simulink library "m3_common_lib"  (R2021b)
settings: Solver=ode45  StartTime=0.0  StopTime=10.0  RelTol=1e-3
undefined symbols (not defined in the file or in its folder): ACCEL_PRE_MULT, APDT_SrvcMgr_IRVHVDCSubFcnReq, C_C1GearNumbers, C_C1GearRatios, C_Calibration, C_DitherWaveform, C_GearOffset, C_GearRatioIn, C_GearRatioInverseOut, C_GearRatioOut, CLUTCH_INNER_LOOP_UPDATE_RATE, CONSTANT, DEGRADED_MODE_SIZE, Dem_EventStatusType, DiscIntNeverNeededParam, F_FAULT_ENUM, F_NOFAULT, F_OUTOFRANGE, F_RATELIMIT, FALSE, FMI14_SPECIAL_INSTRUCTIONS, FMI20_DATA_DRIFTED_HIGH, FMI21_DATA_DRIFTED_LOW, FMI29_RESERVED_FOR_SAE_ASSIGNMENT, FMI30_RESERVED_FOR_SAE_ASSIGNMENT, FMI31_CONDITION_EXISTS, FMI32_NO_FAULT, IC, k_accel, k_mean, MAX_UINT32, MEAN_PRE_MULT, NTriggers, QLTY_SIGNAL_FAILED, QLTY_SIGNAL_FULLY_FUNCTION, QLTY_SIGNAL_SUBSTITUTED_BY_1ST_CHOICE, QLTY_SIGNAL_SUBSTITUTED_BY_2ND_CHOICE, QLTY_SIGNAL_SUBSTITUTED_BY_3RD_CHOICE, QLTY_SIGNAL_SUBSTITUTED_BY_4TH_CHOICE, SAMPLE_TIME_100us, simin, T_TestPoint, TF_FALSE, TF_TRUE, TimeStep, TRUE, WORKSPACE_UPDATE_RATE, Zero, ZERO
libraries: $bdroot x121, simulink x23, simulink_extras x4, MBD_EPS_Local_Blockset x4
(part 1 of 10)
Description:
  | Common library
  | 
  | 
  | 
  | 
  | 
  | 
  | 
  | 
  | 
  | 
  | 
  | 
  | 
  | 
  | 
  | 
  | 
  | 
  | 
  | 
  | 
  | 
  | 
  | 
  | 
  | 
  | 
  | 
  | 
  | 
  | 
  | 
  | 
  | 
  | 
  | 
  | 
  | 
  | 
  | 
  | 
  | 
  | Utility functions useful for embedded control applications.
settings Model: Creator=George Brunemann  LastModifiedBy=E0644758
settings Model: ModifiedComment=|
  | E0072681 -- Fri Jan 08 10:38:41 2010 -- Version 2.15
  | Merged change to cmd-fbk block
settings Model: ModifiedHistory=|
  | E0072681 -- Fri Jan 08 10:38:41 2010 -- Version 2.15
  | Merged change to cmd-fbk block
  | 
  | E0072681 -- Fri Jan 08 10:38:41 2010 -- Version 2.15
  | Merged change to cmd-fbk block
  | 
  | E0072681 -- Fri Jan 08 10:38:27 2010 -- Version 2.14
  | 
  | 
  | E0072118 -- Tue Jan 05 16:47:56 2010 -- Version 2.13
  | 
  | 
  | E0072118 -- Tue Jan 05 16:43:14 2010 -- Version 2.12
  | 
  | 
  | E0072118 -- Fri Dec 18 15:21:16 2009 -- Version 2.11
  | 
  | 
  | E0072118 -- Fri Dec 18 11:28:11 2009 -- Version 2.10
  | 
  | 
  | E0072118 -- Fri Dec 18 11:22:41 2009 -- Version 2.9
  | 
  | 
  | E0072118 -- Fri Dec 18 11:10:11 2009 -- Version 2.8
  | 
  | 
  | E0072118 -- Tue Dec 15 11:02:29 2009 -- Version 2.7
  | 
  | 
  | e0072681 -- Fri Nov 20 14:24:13 2009 -- Version 2.6
  | 
  | 
  | e0072681 -- Fri Nov 20 14:05:16 2009 -- Version 2.5
  | 
  | 
  | E0072681 -- Fri Nov 13 14:35:41 2009 -- Version 2.4
  | 
  | 
  | E0072681 -- Fri Nov 13 11:01:17 2009 -- Version 2.3
  | Added new diagnostic blocks
  | 
  | E0072681 -- Tue Oct 27 17:06:03 2009 -- Version 2.2
  | Changed names on ETP and ETPWT
  | 
  | E0072681 -- Tue Oct 27 15:45:40 2009 -- Version 2.1
  | Merged ETP and ETPWT blocks with IC's into Arbiter library
  | 
  | $Author: allison $ -- $Date: 2006/06/13 14:35:43 $ -- Version $Revision: 1.69 $
settings SolverCC: AlgebraicLoopSolver=TrustRegion
settings DataIOCC: LimitDataPoints=on  SaveFormat=Array  SignalLoggingSaveFormat=ModelDataLogs  ReturnWorkspaceOutputs=off
settings OptimizationCC: BlockReduction=off  BooleanDataType=off  ExpressionDepthLimit=2147483647  LifeSpan=inf
settings DebuggingCC: SaveWithParameterizedLinksMsg=none  UnderspecifiedInitializationDetection=Classic  MergeDetectMultiDrivingBlocksExec=none  SignalResolutionControl=TryResolveAllWithWarning  MultiTaskCondExecSysMsg=none  FcnCallInpInsideContextMsg=warning  StateNameClashWarn=warning  SFUnexpectedBacktrackingDiag=warning  SFNoUnconditionalDefaultTransitionDiag=warning  SFExecutionAtInitializationDiag=none  SFMachineParentedDataDiag=warning  ArithmeticOperatorsInVariantConditions=warning
settings HardwareCC: ProdBitPerPointer=32  ProdBitPerSizeT=32  ProdBitPerPtrDiffT=32  ProdLargestAtomicFloat=None  ProdIntDivRoundTo=Undefined  ProdEndianess=Unspecified  ProdWordSize=32  ProdHWDeviceType=32-bit Generic  TargetUnknown=on
settings ModelReferenceCC: PropagateSignalLabelsOutOfModel=off
settings SFSimCC: SimCustomHeaderCode="#include \"DiagDebounce.h\""  SimUserSources=DiagDebounce.c  CustomCodeUndefinedFunction=UseInterfaceOnly
settings RTWCC: RTWUseSimCustomCode=on  CustomHeaderCode="#include \"DiagDebounce.h\""  CustomSource=DiagDebounce.c
settings CodeAppCC: StateflowObjectComments=on
settings GRTTargetCC: TargetLangStandard=C89/C90 (ANSI)  CombineOutputUpdateFcns=off  GRTInterface=on
settings ConfigComp: CovMetricSettings=dw  CovSaveCumulativeToWorkspaceVar=on  CovSaveSingleToWorkspaceVar=on  CovExternalEMLEnable=off

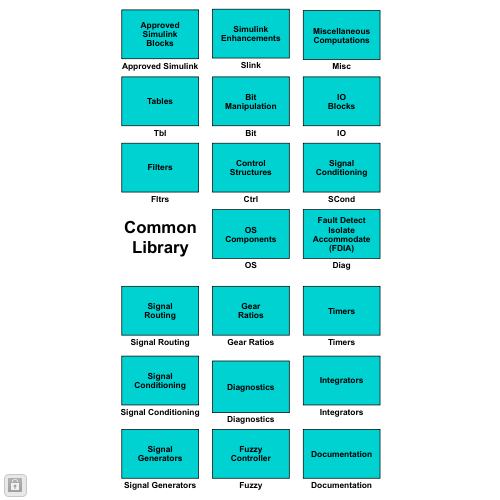
[thumbnail: Simulink's stored preview of the top-level diagram]
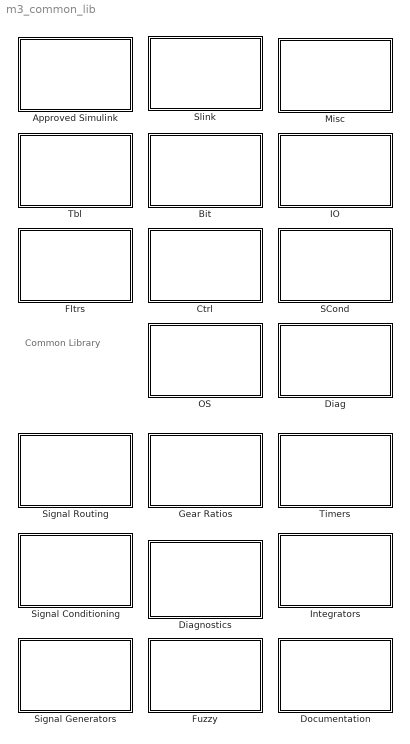
== system m3_common_lib ==
  note: Common
      | Library
  Approved Simulink : Subsystem
      mask Display: disp('Approved\nSimulink\nBlocks')
  Bit : Subsystem
      mask Display: disp('Bit\nManipulation')
  Ctrl : Subsystem
      mask Display: disp('Control\nStructures')
  Diag : Subsystem
      mask Display: disp('Fault Detect\nIsolate\nAccommodate\n(FDIA)')
  Diagnostics : Subsystem
      mask Display: disp('Diagnostics')
  Documentation : Subsystem
      mask Display: disp('Documentation')
  Fltrs : Subsystem
      mask Display: disp('Filters')
  Fuzzy : Subsystem
      mask Display: disp('Fuzzy\nController')
  Gear Ratios : Subsystem
      mask Display: disp('Gear\nRatios')
  IO : Subsystem
      mask Display: disp('IO\nBlocks')
  Integrators : Subsystem
      mask Display: disp('Integrators')
  Misc : Subsystem
      mask Display: disp('Miscellaneous\nComputations')
  OS : Subsystem
      mask Display: disp('OS\nComponents')
  SCond : Subsystem
      mask Display: disp('Signal\nConditioning')
  Signal Conditioning : Subsystem
      mask Display: disp('Signal\nConditioning')
  Signal Generators : Subsystem
      mask Display: disp('Signal\nGenerators')
  Signal Routing : Subsystem
      mask Display: disp('Signal\nRouting')
  Slink : Subsystem
      mask Display: disp('Simulink\nEnhancements')
  Tbl : Subsystem
      mask Display: disp('Tables')
  Timers : Subsystem
      mask Display: disp('Timers')

== system m3_common_lib/Approved Simulink ==
  note: Unit Tested and Approved Simulink Components
  Basic IO : Subsystem
      mask Display: disp('Basic\nInput/Output')
  Discrete And Discontinuities : Subsystem
      mask Display: disp('Discrete')
  Flip Flops : Subsystem
      mask Display: disp('Flip Flops')
  Grouping : Subsystem
      mask Display: disp('Bus and\nMux')
  Math And Logic : Subsystem
      mask Display: disp('Math Operations')
  Signal Attributes : Subsystem
      mask Display: disp('Signal Attributes')
  SubSys Triggers : Subsystem  TreatAsAtomicUnit=on
      mask Display: disp('Subsystem\nEnable and\nTriggers')

== system m3_common_lib/Bit ==
  note: Bit Manipulation
  Bit Operator : Subsystem  mask(CL Bit Operator){Pack=Bit Unpack, DType=UINT8}
      mask prompts: Pack "Binary Operation"; DType "Data Type"
      mask help:
      | Pack or unpack binary data
      |
      | Input and Output vary with mask parameter settings.
      |
      | NgEK, Inc.
      mask init:
      | bit_morph
      mask Help: web(which(['common_lib1.html']))
      mask TypeOptions Pack: Bit Unpack | Bit Pack
      mask TypeOptions DType: UINT8 | UINT16 | UINT32
      mask Display:
      | patch([0.3 0.3 0.7 0.7], [0.35 0.65 0.65 0.35], [255/255 127/255 255/255])
      | disp('Bit\nUnpacker');
      | 
      | port_label('input',1,'Input');
      | port_label('output',1,'Bit 7');
      | port_label('output',2,'Bit 6');
      | port_label('output',3,'Bit 5');
      | port_label('output',4,'Bit 4');
      | port_label('output',5,'Bit 3');
      | port_label('output',6,'Bit 2');
      | port_label('output',7,'Bit 1');
      | port_label('output',8,'Bit 0');
  uint16 Bit Pack : Stateflow chart  TreatAsAtomicUnit=on
  uint16 Bit Unpack : Stateflow chart  TreatAsAtomicUnit=on
  uint8 Bit Pack : Stateflow chart  TreatAsAtomicUnit=on
  uint8 Bit Unpack : Stateflow chart  TreatAsAtomicUnit=on

== system m3_common_lib/Ctrl ==
  note: Control Structures
  Derivative : Subsystem  RTWFcnName=DER  mask(CL Derivative){TimeStep=[]}
      mask prompts: TimeStep "Time Step"
      mask help:
      | Derivative with low pass filtering.  Outputs zero when reset is held, limited to the upper and lower limit inputs.
      |
      | X(1) = input
      | X(2) = low pass cutoff frequency
      | X(3) = upper limit
      | X(4) = lower limit
      | X(5) = reset
      |
      | Y(1) = output
      |
      | Time step is entered via mask parameter.
      | NgEK, Inc.
      mask init:
      | %switch class(TimeStep)
      | % case ('double')
      | %    Zero        = double( 0.0);
      | %    One         = double( 1.0);
      | % case ('single')
      |      Zero        = single( 0.0);
      |      One         = single( 1.0);
      | %end
      | Ts = single(TimeStep);
      settings: RTWFcnNameOpts=User specified  RTWFileNameOpts=Use function name
      mask Help: web(which(['common_lib2.html']))
      mask Display:
      | patch([0.3 0.3 0.7 0.7], [0.35 0.65 0.65 0.35], [255/255 127/255 255/255])
      | disp('Derivative')
      | port_label('input', 1, 'input')
      | port_label('input', 2, 'cutoff')
      | port_label('input', 3, 'ulim')
      | port_label('input', 4, 'llim')
      | port_label('input', 5, 'reset?')
      | port_label('output', 1, 'output')
  Dither : Subsystem  mask(CL Dither){TimeStep=[]}
      mask prompts: TimeStep "Time Step"
      mask help:
      | Output a rectangular dither signal of specified amplitude and frequency.
      | A first order filter of specified time constant is applied to smooth transitions.
      |
      | X(1) = amplitude
      | X(2) = frequency
      | X(3) = filter time constant
      |
      | Y(1) = output
      |
      | Time step is entered via mask parameter.
      | NgEK, Inc.
      mask init:
      | h = [gcb '/Data Type Conversion'];
      | 
      | %switch class(TimeStep)
      | %   case ('double')
      | %      MinusOne    = double(-1.0);
      | %      Zero        = double( 0.0);
      | %      One         = double( 1.0);
      | %      Two         = double( 2.0);
      | %      ZeroFive    = double( 0.5);
      | %      lim         = double(4e-5);
      | %      set_param(h, 'DataType','double');
      | %   case ('single')
      |        MinusOne    = single(-1.0);
      |        Zero        = single( 0.0);
      |        One         = single( 1.0);
      |        Two         = single( 2.0);
      |        ZeroFive    = single( 0.5);
      |        lim         = single(4e-5);
      |        set_param(h, 'DataType','single');
      | %end;
      mask Help: web(which(['common_lib8.html']))
      mask Display:
      | patch([0.375 0.375 0.625 0.625], [0.35 0.65 0.65 0.35], [255/255 127/255 255/255])
      | disp('Dither')
      | port_label('input', 1, 'amplitude')
      | port_label('input', 2, 'frequency')
      | port_label('input', 3, 'tau')
      | port_label('output', 1, 'output')
  Dither w Reset : Subsystem  mask(CL Dither with Reset){TimeStep=[]}
      mask prompts: TimeStep "Time Step"
      mask help:
      | Output a rectangular dither signal of specified amplitude and frequency.
      | A first order filter of specified time constant is applied to smooth transitions.
      |
      | X(1) = amplitude
      | X(2) = frequency
      | X(3) = filter time constant
      |
      | Y(1) = output
      | Y(2) = reset (switched output)
      |
      | Time step is entered via mask parameter.
      | NgEK, Inc.
      mask init: same as m3_common_lib/Ctrl/Dither
      mask Help: web(which(['common_lib9.html']))
      mask Display:
      | patch([0.375 0.375 0.625 0.625], [0.35 0.65 0.65 0.35], [255/255 127/255 255/255])
      | disp('Dither')
      | port_label('input', 1, 'amplitude')
      | port_label('input', 2, 'frequency')
      | port_label('input', 3, 'tau')
      | port_label('output', 1, 'output')
      | port_label('output', 2, 'reset')
  Integrator : Subsystem  TreatAsAtomicUnit=on  RTWFcnName=INTEGRATOR  mask(CL Integrator){TimeStep=SAMPLE_TIME_100us, IC=single(0)}
      mask prompts: TimeStep "Time Step"; IC "Initial Condition"
      mask help:
      | Determine the integral of the input.
      | If reset is true (1), the integrator is set to the reset condition input.
      |
      | X(1) = input
      | X(2) = upper limit
      | X(3) = lower limit
      | X(4) = reset condition
      | X(5) = reset
      |
      | Y(1) = output
      |
      | Time step is entered via mask parameter.
      | Initial condition is entered via mask parameter.
      |
      | NgEK, Inc.
      settings: RTWFcnNameOpts=User specified  RTWFileNameOpts=Use function name
      mask Help: web(which(['common_lib3.html']))
      mask Display:
      | patch([0.3 0.3 0.7 0.7], [0.35 0.65 0.65 0.35], [255/255 127/255 255/255])
      | disp('Integrator')
      | port_label('input', 1, 'input')
      | port_label('input', 2, 'ulim')
      | port_label('input', 3, 'llim')
      | port_label('input', 4, 'reset_cond')
      | port_label('input', 5, 'reset?')
      | port_label('output', 1, 'output')
  PIDgov : Subsystem  mask(CL PID Governor){TimeStep=, MaxInt=, MinInt=, MaxDrv=, MinDrv=, Tol=, IC=}
      mask prompts: TimeStep "Time Step"; MaxInt "Maximum Integrator Value"; MinInt "Minimum Integrator Value"; MaxDrv "Maximum Derivative Value"; MinDrv "Minimum Derivative Value"; Tol "Tolerance"; IC "Initial Condition"
      mask help:
      | Proportional, integral, and derivative governor with anti-windup.
      | Reset sets integral to zero.
      |
      | X(1) = input
      | X(2) = proportional gain
      | X(3) = integral gain
      | X(4) = derivative gain
      | X(5) = low pass cutoff frequency
      | X(6) = controller output upper limit
      | X(7) = controller output lower limit
      | X(8) = reset
      |
      | Y(1) = output
      |
      | Min and max integrator and derivative limits are entered via mask.
      | Time step is entered via mask parameter.
      | Tolerance for detecting saturation is entered via mask.
      | Initial condition is entered via mask.
      |
      | NgEK, Inc.
      mask init:
      | %switch class(TimeStep)
      | %   case ('double')
      | %      Zero        = double( 0.0);
      | %   case ('single')
      |        Zero        = single( 0.0);
      | %end;
      mask Help: web(which(['common_lib6.html']))
      mask Display:
      | patch([0.35 0.35 0.65 0.65], [0.4 0.6 0.6 0.4], [255/255 127/255 255/255])
      | disp('PID gov')
      | port_label('input', 1, 'error')
      | port_label('input', 2, 'p_gain')
      | port_label('input', 3, 'i_gain')
      | port_label('input', 4, 'd_gain')
      | port_label('input', 5, 'cutoff')
      | port_label('input', 6, 'ulim')
      | port_label('input', 7, 'llim')
      | port_label('input', 8, 'reset?')
      | port_label('output', 1, 'output')
  PIDgov w Preset : Subsystem  mask(CL PID Governor with Preset){TimeStep=0.010, MaxInt=1000, MinInt=-1000, MaxDrv=1000, MinDrv=-1000, Tol=1e-6, IC=0.0}
      mask prompts: TimeStep "Time Step"; MaxInt "Maximum Integrator Value"; MinInt "Minimum Integrator Value"; MaxDrv "Maximum Derivative Value"; MinDrv "Minimum Derivative Value"; Tol "Tolerance"; IC "Initial Condition"
      mask help:
      | Proportional plus Integral Governor with anti-windup and integrator preset.
      |
      | Preset sets output to "preset" and resets integrator to achieve that output.
      | Reset sets integral and output to zero.
      |
      | X(1) = input
      | X(2) = proportional gain
      | X(3) = integral gain
      | X(4) = derivative gain
      | X(5) = low pass cutoff frequency
      | X(6) = controller output upper limit
      | X(7) = controller output lower limit
      | X(8) = preset value
      | X(9) = preset
      | X(10) = reset
      |
      | Y(1) = output
      |
      | Min and max integrator and derivative limits are entered via mask.
      | Time step is entered via mask parameter.
      | Tolerance for detecting saturation is entered via mask.
      | Initial condition is entered via mask.
      |
      | NgEK, Inc.
      mask init:
      | %switch class(TimeStep)
      | %   case ('double')
      | %      Zero        = double( 0.0);
      | %   case ('single')
      |        Zero        = single( 0.0);
      | %end;
      mask Help: web(which(['common_lib7.html']))
      mask Display:
      | patch([0.35 0.35 0.65 0.65], [0.4 0.6 0.6 0.4], [255/255 127/255 255/255])
      | disp('PID gov')
      | port_label('input', 1, 'error')
      | port_label('input', 2, 'p_gain')
      | port_label('input', 3, 'i_gain')
      | port_label('input', 4, 'd_gain')
      | port_label('input', 5, 'cutoff')
      | port_label('input', 6, 'ulim')
      | port_label('input', 7, 'llim')
      | port_label('input', 8, 'preset')
      | port_label('input', 9, 'preset?')
      | port_label('input', 10, 'reset?')
      | port_label('output', 1, 'output')
  PIgov : Subsystem  mask(CL PI Governor){TimeStep=, MaxInt=, MinInt=, Tol=, IC=}
      mask prompts: TimeStep "Time Step"; MaxInt "Maximum Integrator Value"; MinInt "Minimum Integrator Value"; Tol "Tolerance"; IC "Initial Condition"
      mask help:
      | Proportional plus integral governor with anti-windup.
      | Reset sets integral to zero.
      |
      | X(1) = input
      | X(2) = proportional gain
      | X(3) = integral gain
      | X(4) = controller output upper limit
      | X(5) = controller output lower limit
      | X(6) = reset
      |
      | Y(1) = output
      |
      | Time step for integrator is entered via mask.
      | Min and max integrator limits are entered via mask.
      | Tolerance for detecting saturation is entered via mask.
      | Initial condition is entered via mask.
      |
      | NgEK, Inc.
      mask init:
      | %switch class(TimeStep)
      | %   case ('double')
      | %      Zero        = double( 0.0);
      | %   case ('single')
      |        Zero        = single( 0.0);
      | %end;
      mask Help: web(which(['common_lib4.html']))
      mask Display:
      | patch([0.35 0.35 0.65 0.65], [0.4 0.6 0.6 0.4], [255/255 127/255 255/255])
      | disp('PI gov')
      | port_label('input', 1, 'error')
      | port_label('input', 2, 'p_gain')
      | port_label('input', 3, 'i_gain')
      | port_label('input', 4, 'ulim')
      | port_label('input', 5, 'llim')
      | port_label('input', 6, 'reset?')
      | port_label('output', 1, 'output')
  PIgov w Preset : Subsystem  mask(CL PI Governor with Preset){TimeStep=, MaxInt=, MinInt=, Tol=, IC=}
      mask prompts: TimeStep "Time Step"; MaxInt "Maximum Integrator Value"; MinInt "Minimum Integrator Value"; Tol "Tolerance"; IC "Initial Condition"
      mask help:
      | Proportional plus integral governor with anti-windup and integrator preset.
      |
      | Preset sets output to "preset" and resets integrator to achieve that output.
      | Reset sets integrator and output to zero.
      |
      | X(1) = input
      | X(2) = proportional gain
      | X(3) = integral gain
      | X(4) = controller output upper limit
      | X(5) = controller output lower limit
      | X(6) = output preset
      | X(7) = preset
      | X(8) = reset
      |
      | Y(1) = output
      |
      | Time step for integrator is entered via mask.
      | Min and max integrator limits are entered via mask.
      | Tolerance for detecting saturation is entered via mask.
      | Initial condition is entered via mask.
      |
      | NgEK, Inc.
      mask init:
      | %switch class(TimeStep)
      | %   case ('double')
      | %      Zero        = double( 0.0);
      | %   case ('single')
      |        Zero        = single( 0.0);
      | %end;
      mask Help: web(which(['common_lib5.html']))
      mask Display:
      | patch([0.35 0.35 0.65 0.65], [0.4 0.6 0.6 0.4], [255/255 127/255 255/255])
      | disp('PI gov')
      | port_label('input', 1, 'error')
      | port_label('input', 2, 'p_gain')
      | port_label('input', 3, 'i_gain')
      | port_label('input', 4, 'ulim')
      | port_label('input', 5, 'llim')
      | port_label('input', 6, 'preset')
      | port_label('input', 7, 'preset?')
      | port_label('input', 8, 'reset?')
      | port_label('output', 1, 'output')
  Ramp : Subsystem  TreatAsAtomicUnit=on  RTWFcnName=RAMP  mask(CL ramp){TimeStep=[]}
      mask prompts: TimeStep "Time Step"
      mask help:
      | Ramp from A to B over time interval C
      | If reset is true (1), the output is held at the A input.
      |
      | X(1) = starting point for ramp
      | X(2) = ending point for ramp
      | X(3) = time interval for ramp
      | X(4) = reset
      |
      | Y(1) = output
      |
      | Time step is entered via mask parameter.
      |
      | NgEK, Inc.
      mask init:
      | %switch class(TimeStep)
      | %   case ('double')
      | %      Zero        = double( 0.0);
      | %   case ('single')
      |        Zero        = single( 0.0);
      | %end;
      settings: RTWFcnNameOpts=User specified  RTWFileNameOpts=Use function name
      mask Help: web(which(['common_lib50.html']))
      mask Display:
      | patch([0.2 0.2 0.8 0.8], [0.2 0.8 0.8 0.2], [255/255 127/255 255/255])
      | 
      | plot([0.25 0.4 0.6 .75],[.25 .25 .75 .75])
      | 
      | text(.3,.35,'A');text(.65,.65,'B');text(.5,.4,'C')
      | 
      | port_label('input', 1, 'A')
      | port_label('input', 2, 'B')
      | port_label('input', 3, 'C')
      | port_label('input', 4, 'reset?')
      | port_label('output', 1, 'out')
  Subsystem : Subsystem  TreatAsAtomicUnit=on  RTWFcnName=HistogramCntr
      settings: RTWFcnNameOpts=User specified  RTWFileNameOpts=Use function name
  Trajectory : Subsystem  mask(CL Trajectory){TimeStep=, StartRLimIn=, StartRLimOut=, FinalRLimIn=, FinalRLimOut=}
      mask prompts: TimeStep "Time Step"; StartRLimIn "Start Rate Limit Input"; StartRLimOut "Start Rate Limit Output"; FinalRLimIn "Final Rate Limit Input"; FinalRLimOut "Final Rate Limit Output"
      mask help:
      | Control the shape from start_value to final_value using a table of filter tau versus time.
      |
      | The weight stretches the trajectory for values > 1.
      | The weight compresses the trajectory for values <1.
      |
      | X(1)=start_value
      | X(2)=final_value
      | X(3)=weight
      | X(4)=start flag
      |
      | Y(1)=output
      |
      | Update rate, vector of time inputs and tau outputs is entered via mask parameter.
      | NgEK, Inc.
      mask init:
      | %switch class(TimeStep)
      | %   case ('double')
      | %      Zero       = double( 0.0);
      | %      MinusOne   = double(-1.0);
      | %      tol        = double(1e-6);
      | %   case ('single')
      |        Zero       = single( 0.0);
      |        MinusOne   = single(-1.0);
      |        tol       = single(1e-6);
      | %end;
      mask Help: web(which(['common_lib10.html']))
      mask Display:
      | patch([0.4 0.4 0.6 0.6], [0.35 0.65 0.65 0.35], [255/255 127/255 255/255])
      | disp('Traj')
      | port_label('input', 1, 'start_value')
      | port_label('input', 2, 'final_value')
      | port_label('input', 3, 'start_weight')
      | port_label('input', 4, 'final_weight')
      | port_label('input', 5, 'start?')
      | port_label('output', 1, 'output')

== system m3_common_lib/Diag ==
  note: Diagnostics
  CL MinMax Capture : Subsystem  RTWFcnName=MinMaxCap  mask(CL Max Capture){CaptureType=Min, InDataType=single}
      mask prompts: CaptureType "Capture Function"; InDataType "Input DataType"
      mask help:
      | Capture the maximum/minimum value for the input.
      |
      | x(1) = input
      | x(2) = hold?        (hold current max/min value)
      | x(3) = reset?       (reset the output to initial value)
      |
      | y(1) = output
      |
      | The capture function and Input signal datatype are entered via mask parameters.
      |
      | Eaton Controls Engineering COE, 2010.
      mask init:
      | % Change the relational operation and outport label
      | h_input = [gcb '/Relational Operator'];
      | 
      | switch (get_param(gcb,'CaptureType'))
      |     case('Min')
      |        set_param(h_input,'Operator','<');
      |        initvalue = double(999999999999);
      |     case('Max')
      |         set_param(h_input,'Operator','>');
      |         initvalue = double(-999999999999);
      | end;
      | 
      | % Set the Init value to the appropriate value
      | % value for the data type
      | 
      | switch (get_param(gcb,'InDataType'))
      |    case ('double')
      |         InitValue    = double(initvalue);
      |    case ('single')
      |         InitValue    = single(initvalue);
      |    case ('uint32')
      |         InitValue    = uint32(initvalue);
      |    case ('int32')
      |         InitValue    = int32(initvalue);
      |    case ('uint16')
      |         InitValue    = uint16(initvalue);
      |    case ('int16')
      |         InitValue    = int16(initvalue);
      |    case ('uint8')
      |         InitValue    = uint8(initvalue);
      |    case ('int8')
      |         InitValue    = int8(initvalue); 
      | end;
      settings: RTWFcnNameOpts=User specified  RTWFileNameOpts=Use function name
      mask TypeOptions CaptureType: Min | Max
      mask TypeOptions InDataType: double | single | uint32 | int32 | uint16 | int16 | uint8 | int8
      mask Display:
      | patch([0.3 0.3 0.7 0.7],[0.4 0.6 0.6 0.4],[255/255 127/255 255/255])
      | 
      | disp([get_param(gcb,'CaptureType') ' Capture'])
      | 
      | port_label('input', 1, 'input')
      | port_label('input', 2, 'hold?')
      | port_label('input', 3, 'reset?')
      | port_label('output', 1, [get_param(gcb,'CaptureType') ' Value'])
  Command Feedback Test : Subsystem  TreatAsAtomicUnit=on  RTWFcnName=CFT  mask(CL Command Feedback Test){TimeStep=[]}
      mask prompts: TimeStep "Time Step (seconds)"
      mask help:
      | System level check to test if control command is being achieved.
      |
      | During "steady state", check that cmd - fbk  < error_lim
      | Error must occur for error_time seconds before fault is set.
      | Error must not occur for error_time seconds before fault is cleared.
      |
      | "Steady state" is defined as:
      |   command is within tau_lim of filtered command for tau_time
      |
      | NgEK, Inc.
      mask init:
      | %switch class(TimeStep)
      | %   case ('double')
      | %      Zero     = double( 0.0);
      | %      One      = double( 1.0);
      | %      MinusOne = double(-1.0);
      | %   case ('single')
      |        Zero     = single( 0.0);
      |        One      = single( 1.0);
      |        MinusOne = single(-1.0);
      | %end;
      | Ts = single(TimeStep);
      settings: RTWFcnNameOpts=User specified  RTWFileNameOpts=Use function name
      mask Help: web(which(['common_lib11.html']))
      mask Display:
      | patch([0.3 0.3 0.7 0.7], [0.4 0.6 0.6 0.4], [255/255 127/255 255/255]);
      | disp('Cmd-Fbk');
  Fault Counter : Subsystem  RTWFcnName=FLTCNTR  mask(FL Counter){DATATYPE=int16}
      mask prompts: DATATYPE "Counter datatype"
      mask help:
      | Generic fault counter block.
      | Counts up by up_count when fl? is true
      | Counts down by down_count when fl? is false.
      | Sets fc? true if fc_level is reached and clears fc? if zero is reached.
      |
      | X(1) = fault flag
      | X(2) = up count value (positive number)
      | X(3) = down count value (negative number)
      | X(4) = fault code active level
      | X(5) = reset fault code to false and count to zero
      |
      | Y(1) = fault code active flag
      |
      | Initial condition is entered via mask.
      | NgEK, Inc.
      mask init:
      | switch DATATYPE
      |     case (1) %('double')
      |         ZERO     = double(0.0);
      |   case (2) %('single')
      |         ZERO     = single(0.0);
      |   case (3) %('int8')
      |         ZERO     = int8(0.0);
      |     case (4) %('int16')
      |        ZERO     = int16(0.0);
      |    case (5) %('int32')
      |        ZERO     = int32(0.0);
      | end;
      | 
      | strDtype = get_param(gcb,'DATATYPE');
      | %set_param([gcb '/DTC2'],'OutDataTypeStr',strDtype);
      | set_param([gcb '/DTC3'],'OutDataTypeStr',strDtype);
      | %set_param([gcb '/DTC4'],'OutDataTypeStr',strDtype);
      settings: RTWFcnNameOpts=User specified  RTWFileNameOpts=Use function name
      mask Help: web(which(['common_lib49.html']))
      mask TypeOptions DATATYPE: double | single | int8 | int16 | int32
      mask Display:
      | patch([0.35 0.35 0.65 0.65], [0.25 0.75 0.75 0.25], [255/255 127/255 255/255])
      | disp('Fault\nCounter')
      | port_label('input', 1, 'fl?')
      | port_label('input', 2, 'true_count')
      | port_label('input', 3, 'false_count')
      | port_label('input', 4, 'fc_level')
      | port_label('input', 5, 'reset?')
      | port_label('output', 1, 'fc?')
  Fault Counter w Hold : Subsystem  mask(FL Counter){DATATYPE=int16}
      mask prompts: DATATYPE "Counter datatype"
      mask help:
      | Generic fault counter block.
      | Freezes count when hold? is true
      | Counts up by up_count when fl? is true
      | Counts down by down_count when fl? is false.
      | Sets fc? true if fc_level is reached and clears fc? if zero is reached.
      |
      | X(1) = fault flag
      | X(2) = hold flag
      | X(3) = up count value (positive number)
      | X(4) = down count value (negative number)
      | X(5) = fault code active level
      | X(6) = reset fault code to false and count to zero
      |
      | Y(1) = fault code active flag
      |
      | Initial condition is entered via mask.
      | NgEK, Inc.
      mask init:
      | switch DATATYPE
      |     case (1) %('double')
      |         ZERO     = double(0.0);
      |   case (2) %('single')
      |         ZERO     = single(0.0);
      |   case (3) %('int8')
      |         ZERO     = int8(0.0);
      |     case (4) %('int16')
      |        ZERO     = int16(0.0);
      |    case (5) %('int32')
      |        ZERO     = int32(0.0);
      | end;
      mask Help: web(which(['common_lib49.html']))
      mask TypeOptions DATATYPE: double | single | int8 | int16 | int32
      mask Display:
      | patch([0.35 0.35 0.65 0.65], [0.25 0.75 0.75 0.25], [255/255 127/255 255/255])
      | disp('Fault\nCounter\nw/Hold')
      | port_label('input', 1, 'fl?')
      | port_label('input', 2, 'hold?')
      | port_label('input', 3, 'true_count')
      | port_label('input', 4, 'false_count')
      | port_label('input', 5, 'fc_level')
      | port_label('input', 6, 'reset?')
      | port_label('output', 1, 'fc?')
  Fault Injection : Subsystem  mask(CL Fault Injection){InitialValue=[]}
      mask prompts: InitialValue "Initial Condition"
      mask help:
      | Used to inject faults on input signals.
      | The gain/offset results in the output = gain*input - offset.
      | Nominal values (no fault) should be:
      |         gain = 1
      |       offset = 0
      |        fl_trigger=FALSE
      |
      | The ulim and llim are applied to the Out Of Range detection.
      |
      | hold is a boolean to hold output at last in range value.
      | fl_trigger is a boolean to trigger a fault flag and hold last in range value.
      mask init:
      | h=[gcb '/Gain and Offset (in)'];
      | 
      | switch class(InitialValue)
      |   case ('int8')
      |      set_param(h, 'MaskValueString','int8');
      |    case ('uint8')
      |         set_param(h, 'MaskValueString','uint8');
      |   case ('int16')
      |         set_param(h, 'MaskValueString','int16');
      |  case ('uint16')
      |        set_param(h, 'MaskValueString','uint16');
      |   case ('single')
      |       set_param(h, 'MaskValueString','single');
      |  case ('double')
      |        set_param(h, 'MaskValueString','double');   
      |   otherwise
      |       set_param(h, 'MaskValueString','single');
      | end
      mask Help: web(which(['common_lib15.html']))
      mask Display:
      | patch([0.30 0.30 0.70 0.70], [0.40 0.60 0.60 0.40], [255/255 127/255 255/255])
      | disp('Fault Inection')
      | port_label('input', 1, 'input')
      | port_label('input', 2, 'gain')
      | port_label('input', 3, 'offset')
      | port_label('input', 4, 'ulim')
      | port_label('input', 5, 'llim')
      | port_label('input', 6, 'hold')
      | port_label('input', 7, 'fl_trigger')
      | port_label('output', 1, 'output')
      | port_label('output', 2, 'hwfl')
  Fault Log : Subsystem  mask(CL Fault Log){EventDataType=uint16, FrameDataType=uint32}
      mask prompts: EventDataType "Events Datatype"; FrameDataType "Frames Datatype"
      mask help:
      | Fault logger.
      | Count number of activations of the fault and the total time the fault has been active
      |
      | X(1) = fault flag
      | X(2) = events state
      | X(3) = frames state
      | X(4) = hold flag (ignore inputs while TRUE)
      |
      | Y(1) = fault count
      | Y(2) = fault active time
      |
      | NgEK, Inc.
      mask init:
      | a = get_param(gcb,'FrameDataType');
      | set_param([gcb '/HWfl_Frames'],'OutDataTypeStr',a);
      | 
      | FRAME_ONE = eval([a '(1)']);
      | FRAME_MAX = intmax(a);
      | FRAME_ZERO = eval([a '(0)']);
      | 
      | a = get_param(gcb,'EventDataType');
      | set_param([gcb '/HWfl_Events'],'OutDataTypeStr',a);
      | 
      | EVENT_ONE = eval([a '(1)']);
      | EVENT_MAX = intmax(a);
      | EVENT_ZERO = eval([a '(0)']);
      mask Help: web(which(['common_lib13.html']))
      mask TypeOptions EventDataType: uint8 | uint16 | uint32
      mask TypeOptions FrameDataType: uint8 | uint16 | uint32
      mask Display:
      | patch([0.3 0.3 0.7 0.7], [0.3 0.7 0.7 0.3], [255/255 127/255 255/255])
      | disp('Fault\nLog')
      | port_label('input',1,'active')
      | port_label('input',2,'events')
      | port_label('input',3,'frames')
      | port_label('input',4,'hold?')
      | port_label('output',1,[get_param(gcb,'EventDataType') ' events'])
      | port_label('output',2,[get_param(gcb,'FrameDataType') ' frames'])
  Fault_Cntr : Subsystem  Tag=HYB_CL  RTWFcnName=FC_FMI_Handler  mask(FL Counter){fc_level=int16(100), up_cnt=int16(100), dn_cnt=int16(-1), fid=F_FAULT_ENUM, amber=false, red=false}
      mask prompts: amber "set_amber_light"; red "set_red_light"
      mask help:
      | Generic fault counter and relay block.
      | Counts up by up_cnt when flg is true
      | Counts down by dn_cnt when flg is false.
      |
      | Once the count reaches fc_level
      | Sets fc_fmi = (fid << 8 || fmi) and
      |  if red,        lights = 2
      |  elseif amber,  lights = 1
      |  else,          lights = 0
      |
      | Clears fc_fmi and lights once the count reaches 0.
      |
      | X(1) = fault flag
      | X(2) = reset fault code to false and count to zero
      | X(3) = failure mode identifier (FMI)
      |
      | Y(1) = (FID and FMI) for active fault
      | Y(2) = light status
      |
      | Counter and FID/FMI are always initialized to zero
      | Eaton, Corp.
      mask init:
      | fc_count = int16(fc_level);
      | dn_count = int16(dn_cnt);
      | up_count = int16(up_cnt);
      | fault_id = uint16(fid);
      | red_light = boolean(red);
      | amber_light = boolean(amber);
      settings: RTWFcnNameOpts=User specified  RTWFileNameOpts=Use function name
      mask Help: web(which(['common_lib49.html']))
      mask Display:
      | patch([0.35 0.35 0.65 0.65], [0.25 0.75 0.75 0.25], [255/255 127/255 255/255])
      | disp(get_param(gcb,'fid'))
      | port_label('input', 1, 'flg')
      | port_label('input', 2, 'rst')
      | port_label('input',3,'fmi')
      | port_label('output', 1, 'fc_fmi')
      | port_label('output',2,'lights')
  Filter w Fault Handler : Subsystem  RTWFcnName=FLTRWROFH  mask(CL Fault Handle){TimeStep=[]}
      mask prompts: TimeStep "Time Step"
      mask help:
      | Fault handler
      |
      | Upon onset of fault, ramp signal up or down to default value over given time.
      | Upon fault clear, switch back to filtered input signal.
      |
      | NgEK, Inc.
      mask init:
      | %switch class(TimeStep)
      | %   case ('double')
      | %      Zero     = double( 0.0);
      | %   case ('single')
      |        Zero     = single( 0.0);
      | %end;
      settings: RTWFcnNameOpts=User specified  RTWFileNameOpts=Use function name
      mask Help: web(which(['common_lib14.html']))
      mask Display:
      | patch([0.30 0.30 0.70 0.70], [0.40 0.60 0.60 0.40], [255/255 127/255 255/255])
      | disp('Filter w/RO\nFault Handler')
      | port_label('input', 1, 'input')
      | port_label('input', 2, 'tau')
      | port_label('input', 3, 'override_value')
      | port_label('input', 4, 'override?')
      | port_label('input', 5, 'reset?')
      | port_label('input', 6, 'default')
      | port_label('input', 7, 'ramp_time')
      | port_label('input', 8, 'fault?')
      | port_label('output', 1, 'output')
  Filter w Fault Handler1 : Subsystem  TreatAsAtomicUnit=on  RTWFcnName=FLTRWFH  mask(CL Fault Handle){TimeStep=[]}
      mask prompts: TimeStep "Time Step"
      mask help:
      | FILTER WITH FAULT HANDLER
      |
      | INPUTS
      | U  = Input signal
      | TC = Time Constant
      | RST = Reset
      | DV = Default Value
      | RT = Ramp Time
      | FLT = Fault
      |
      | OUTPUTS
      | Y = Output signal
      |
      | Upon onset of fault, ramp signal up or down to default value over given time.
      | Upon fault clear, switch back to filtered input signal.
      |
      | NgEK, Inc.
      mask init:
      | switch class(TimeStep)
      |  case ('double')
      |       Zero     = double( 0.0);
      |     case ('single')
      |          Zero     = single( 0.0);
      | end;
      settings: RTWFcnNameOpts=User specified  RTWFileNameOpts=Use function name
      mask Help: web(which(['common_lib14.html']))
      mask Display:
      | patch([0.30 0.30 0.70 0.70], [0.40 0.60 0.60 0.40], [255/255 127/255 255/255])
      | disp('Filter with\nFault Handler')
      | port_label('input', 1, 'U')
      | port_label('input', 2, 'TC')
      | port_label('input', 3, 'RST')
      | port_label('input', 4, 'DV')
      | port_label('input', 5, 'RT')
      | port_label('input', 6, 'FLT')
      | port_label('output', 1, 'Y')
  OOR Fault Detection : Subsystem  TreatAsAtomicUnit=on  RTWFcnName=OOR  mask(CL OOR Fault Detection){InitialValue=[]}
      mask prompts: InitialValue "Initial Value"
      mask help:
      | Out of range fault detection block
      |
      | X(1) = input signal
      | X(2) = upper limit
      | X(3) = lower limit
      | X(4) = external fault flag
      |
      | Y(1) = output
      | Y(2) = fault indication
      | NgEK, Inc.
      settings: RTWFcnNameOpts=User specified  RTWFileNameOpts=Use function name
      mask Help: web(which(['common_lib12.html']))
      mask Display:
      | patch([0.3 0.3 0.7 0.7], [0.35 0.65 0.65 0.35], [255/255 127/255 255/255])
      | disp('OOR')
      | port_label('input',1,'in')
      | port_label('input',2,'ulim')
      | port_label('input',3,'llim')
      | port_label('input',4,'ext_fl?')
      | port_label('output',1,'out')
      | port_label('output',2,'fault?')
  Rate Limit Fault Detection : Subsystem  TreatAsAtomicUnit=on  RTWFcnName=RLIM  mask(CL Rate Limit Fault Detection){IC=0, TimeStep=0}
      mask prompts: IC "Initial Condition"; TimeStep "Update Time"
      mask help:
      | Rate limit fault detection block
      |
      | X(1) = input signal
      | X(2) = rate limit
      | X(3) = external fault flag
      |
      | Y(1) = output
      | Y(2) = fault indication
      | NgEK, Inc.
      mask init:
      | %switch class(TimeStep)
      | %   case ('double')
      | %      Zero     = double(0.0);
      | %   case ('single')
      |        Zero     = single(0.0);
      | %   case ('int8')
      | %      Zero     = int8(0.0);
      | %   case ('int16')
      | %      Zero     = int16(0.0);
      | %   case ('int32')
      | %      Zero     = int32(0.0);
      | %end;
      settings: RTWFcnNameOpts=User specified  RTWFileNameOpts=Use function name
      mask Help: web(which(['common_lib46.html']))
      mask Display:
      | patch([0.3 0.3 0.7 0.7], [0.35 0.65 0.65 0.35], [255/255 127/255 255/255])
      | disp('RLim')
      | port_label('input',1,'in')
      | port_label('input',2,'rlim')
      | port_label('input',3,'ext_fl?')
      | port_label('output',1,'out')
      | port_label('output',2,'fault?')
